simulink model "BicyclePeterCorkePoseReach"  (R2021a)
settings: Solver=VariableStepAuto  StartTime=0.0  StopTime=30  RelTol=1e-3
values from neighbouring files (symbols this model uses):
  accelLim = 1    [BicyclePeterCorkeLineFollowSetup.m]    (also in BicyclePeterCorkePathFollowSetup.m; BicyclePeterCorkePoseReachSetup.m)
  goalPose = [5 5 pi/2]    [BicyclePeterCorkePoseReachSetup.m]
  initPose = [9 5 0]    [BicyclePeterCorkePoseReachSetup.m]
  speedLim = 1    [BicyclePeterCorkeLineFollowSetup.m]    (also in BicyclePeterCorkePathFollowSetup.m; BicyclePeterCorkePoseReachSetup.m)
  steerLim = 1    [BicyclePeterCorkeLineFollowSetup.m]    (also in BicyclePeterCorkePathFollowSetup.m; BicyclePeterCorkePoseReachSetup.m)
  wheelBase = 1    [BicyclePeterCorkeLineFollowSetup.m]    (also in BicyclePeterCorkePathFollowSetup.m; BicyclePeterCorkePoseReachSetup.m)
libraries: simulink x2
settings Model: Creator=guyot  LastModifiedBy=guyot

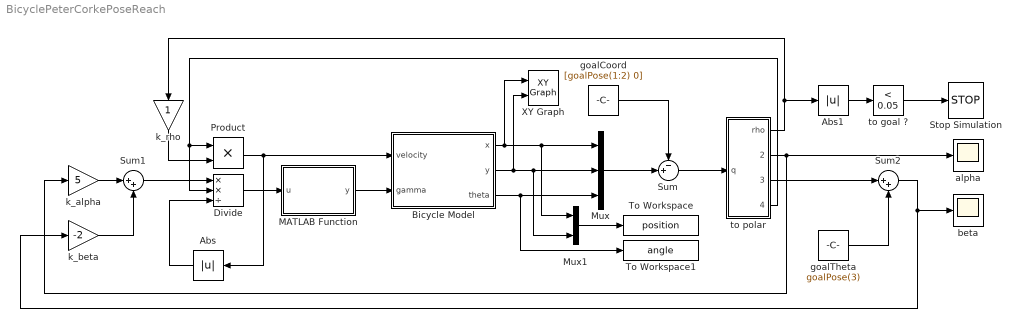
== system BicyclePeterCorkePoseReach ==
  Abs : Abs
  Abs1 : Abs
  Bicycle Model : Subsystem
  Divide : Product  Inputs=**/
  MATLAB Function : MATLAB Function  TreatAsAtomicUnit=on
  Mux : Mux  Inputs=3
  Mux1 : Mux  Inputs=2
  Product : Product
  Stop Simulation : Stop
  Sum : Sum  Inputs=-+|
  Sum1 : Sum  Inputs=|++
  Sum2 : Sum  Inputs=|++
  To Workspace : ToWorkspace  VariableName=position  SaveFormat=Timeseries  SampleTime=-1
  To Workspace1 : ToWorkspace  VariableName=angle  SaveFormat=Timeseries  SampleTime=-1
  XY Graph : simulink/Sinks/XY Graph  xmin=0  xmax=10  ymin=0  ymax=10  st=-1
  alpha : Scope
  beta : Scope
  goalCoord : Constant  Value=[goalPose(1:2) 0]
  goalTheta : Constant  Value=goalPose(3)
  k_alpha : Gain  Gain=5
  k_beta : Gain  Gain=-2
  k_rho : Gain
  to goal ? : simulink/Logic and Bit Operations/Compare To Constant  relop=<  const=0.05  OutDataTypeStr=boolean
  to polar : Subsystem
  wires:
  MATLAB Function/1(y) -> Bicycle Model/2(gamma)
  to goal ?/1 -> Stop Simulation/1
  Product/1 -> Abs/1, Bicycle Model/1(velocity)
  Divide/1 -> MATLAB Function/1(u)
  Bicycle Model/1(x) -> XY Graph/1, Mux1/1, Mux/1
  Bicycle Model/2(y) -> Mux1/2, Mux/2, XY Graph/2
  Bicycle Model/3(theta) -> To Workspace1/1, Mux/3
  goalCoord/1 -> Sum/1
  Mux/1 -> Sum/2
  Sum/1 -> to polar/1(q)
  to polar/1(rho) -> k_rho/1, Abs1/1
  Abs1/1 -> to goal ?/1
  Sum1/1 -> Divide/1
  k_alpha/1 -> Sum1/1
  k_beta/1 -> Sum1/2
  to polar/2(alpha) -> k_alpha/1, alpha/1
  Sum2/1 -> k_beta/1, beta/1
  goalTheta/1 -> Sum2/2
  to polar/3(beta) -> Sum2/1
  to polar/4(direction) -> Divide/2, Product/1
  k_rho/1 -> Product/2
  Abs/1 -> Divide/3
  Mux1/1 -> To Workspace/1

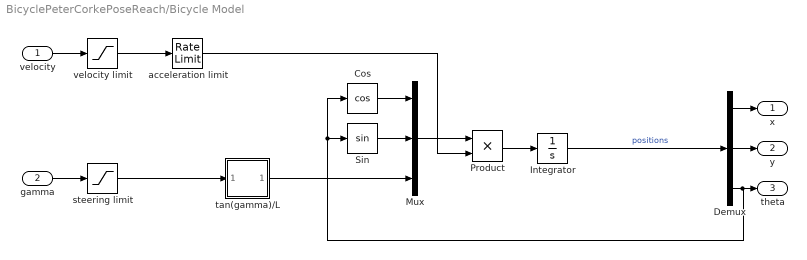
== system BicyclePeterCorkePoseReach/Bicycle Model ==
  velocity : Inport
  gamma : Inport  Port=2
  Cos : Trigonometry  Operator=cos
  Demux : Demux  Outputs=3
  Integrator : Integrator  InitialCondition=initPose
  Mux : Mux  Inputs=3
  Product : Product
  Sin : Trigonometry
  acceleration limit : RateLimiter  RisingSlewLimit=accelLim  FallingSlewLimit=-accelLim  SampleTimeMode=inherited
  steering limit : Saturate  UpperLimit=steerLim  LowerLimit=-steerLim
  tan(gamma)/L : Subsystem
  velocity limit : Saturate  UpperLimit=speedLim  LowerLimit=-speedLim
  x : Outport
  y : Outport  Port=2
  theta : Outport  Port=3
  wires:
  velocity/1 -> velocity limit/1
  velocity limit/1 -> acceleration limit/1
  gamma/1 -> steering limit/1
  steering limit/1 -> tan(gamma)/L/1(In1)
  tan(gamma)/L/1(Out1) -> Mux/3
  Mux/1 -> Product/1
  acceleration limit/1 -> Product/2
  Product/1 -> Integrator/1
  Integrator/1 -> Demux/1  "positions"
  Demux/3 -> Cos/1, Sin/1, theta/1
  Demux/1 -> x/1
  Demux/2 -> y/1
  Cos/1 -> Mux/1
  Sin/1 -> Mux/2

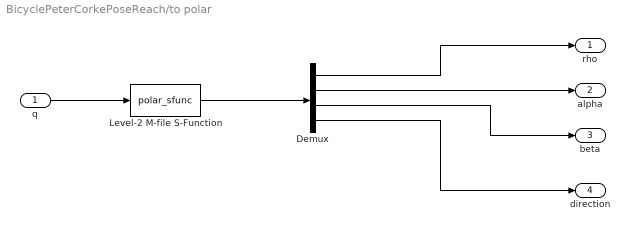
== system BicyclePeterCorkePoseReach/to polar ==
  q : Inport
  Demux : Demux
  Level-2 M-file S-Function : M-S-Function  FunctionName=polar_sfunc
  rho : Outport  VectorParamsAs1DForOutWhenUnconnected=off
  alpha : Outport  Port=2  VectorParamsAs1DForOutWhenUnconnected=off
  beta : Outport  Port=3  VectorParamsAs1DForOutWhenUnconnected=off
  direction : Outport  Port=4  VectorParamsAs1DForOutWhenUnconnected=off
  wires:
  Demux/3 -> beta/1
  Demux/1 -> rho/1
  Demux/2 -> alpha/1
  Demux/4 -> direction/1
  Level-2 M-file S-Function/1 -> Demux/1
  q/1 -> Level-2 M-file S-Function/1

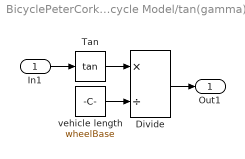
== system BicyclePeterCorkePoseReach/Bicycle Model/tan(gamma)//L ==
  In1 : Inport
  Divide : Product  Inputs=*/
  Tan : Trigonometry  Operator=tan
  vehicle length : Constant  Value=wheelBase
  Out1 : Outport
  wires:
  Tan/1 -> Divide/1
  vehicle length/1 -> Divide/2
  In1/1 -> Tan/1
  Divide/1 -> Out1/1

== matlab function BicyclePeterCorkePoseReach/MATLAB Function ==
  data: u input; y output
function y = arctan(u)

y = atan(u);
